simulink model "W02_pid"  (R2024b)
settings: Solver=ode4  StartTime=0  StopTime=T_final  FixedStep=h  RelTol=1e-3
StopFcn:
  | W02_plot;
values from neighbouring files (symbols this model uses):
  d_filtered = 1    [W02_0_setup.m]
  Kb = 2    [W02_0_setup.m]
  Kd = 4    [W02_0_setup.m]    (also in W02_E_integral.m; W02_I_tuning_by_hand.m = 1)
  Ki = 8    [W02_0_setup.m]
  Kp = 10    [W02_0_setup.m]    (also in W02_D_derivative.m; W02_E_integral.m; W02_I_tuning_by_hand.m = 5*k)
  Nf = 20    [W02_0_setup.m]    (also in W02_G_lowpass_filter.m = Nf(i))
  noise_std = 0    [W02_0_setup.m]
  noise_ts = 0.01    [W02_0_setup.m]
  pid_b = 2    [W02_0_setup.m]
  pid_k = 2    [W02_0_setup.m]
  pid_m = 1    [W02_0_setup.m]
  ref_filter = 0    [W02_0_setup.m]
  ref_Tf = 0.3    [W02_0_setup.m]
  t_step = 1    [W02_0_setup.m]
  tau_max = 1e6    (= 1000000)    [W02_0_setup.m]
  y_step = 1    [W02_0_setup.m]
libraries: slpidlib x1
settings Model: Creator=admin  LastModifiedBy=admin
settings DataIOCC: ReturnWorkspaceOutputs=off

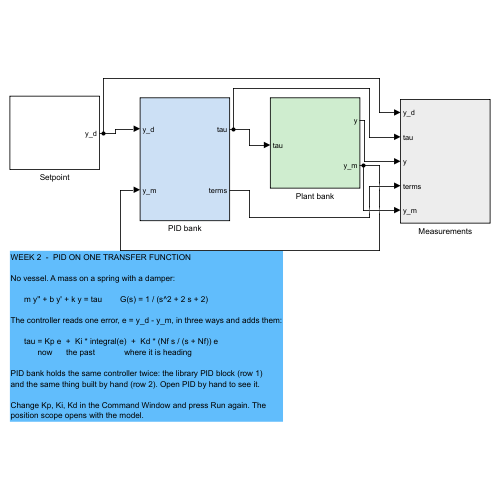
[thumbnail: Simulink's stored preview of the top-level diagram]
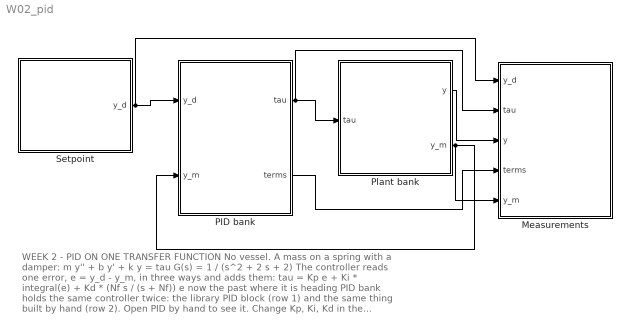
== system W02_pid ==
  note: WEEK 2  -  PID ON ONE TRANSFER FUNCTION
      |
      | No vessel. A mass on a spring with a damper:
      |
      |       m y'' + b y' + k y = tau        G(s) = 1 / (s^2 + 2 s + 2)
      |
      | The controller reads one error, e = y_d - y_m, in three ways and adds them:
      |
      |       tau = Kp e  +  Ki * integral(e)  +  Kd * (Nf s / (s + Nf)) e
      |             now      the past             where it is heading
      |
      | PID bank holds the same controller twice: the library PID block (row 1)
      | and the same thing built by hand (row 2). Open PID by hand to see it.
      |
      | Change Kp, Ki, Kd in the Command Window and press Run again. The
      | position scope opens with the model.
  Measurements : Subsystem
  PID bank : Subsystem
  Plant bank : Subsystem
  Setpoint : Subsystem
  wires:
  Setpoint/1(y_d) -> PID bank/1(y_d), Measurements/1(y_d)
  Plant bank/2(y_m) -> PID bank/2(y_m), Measurements/5(y_m)
  PID bank/1(tau) -> Plant bank/1(tau), Measurements/2(tau)
  Plant bank/1(y) -> Measurements/3(y)
  PID bank/2(terms) -> Measurements/4(terms)

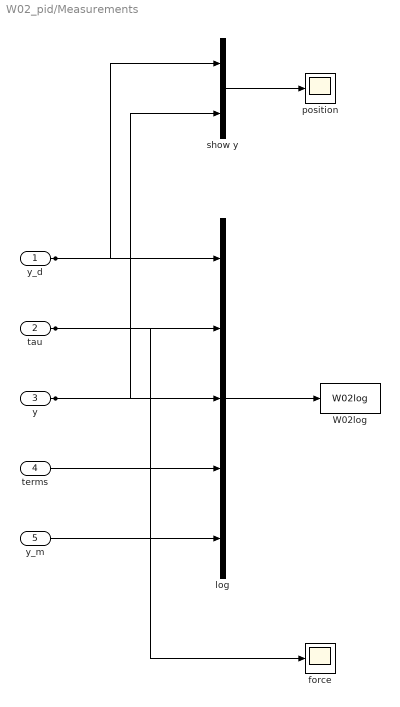
== system W02_pid/Measurements ==
  y_d : Inport
  tau : Inport  Port=2
  y : Inport  Port=3
  terms : Inport  Port=4
  y_m : Inport  Port=5
  W02log : ToWorkspace  VariableName=W02log  SaveFormat=Structure With Time  SampleTime=-1
  force : Scope
  log : Mux  Inputs=5
  position : Scope
  show y : Mux  Inputs=2
  wires:
  y_d/1 -> log/1, show y/1
  tau/1 -> log/2, force/1
  y/1 -> log/3, show y/2
  terms/1 -> log/4
  y_m/1 -> log/5
  log/1 -> W02log/1
  show y/1 -> position/1

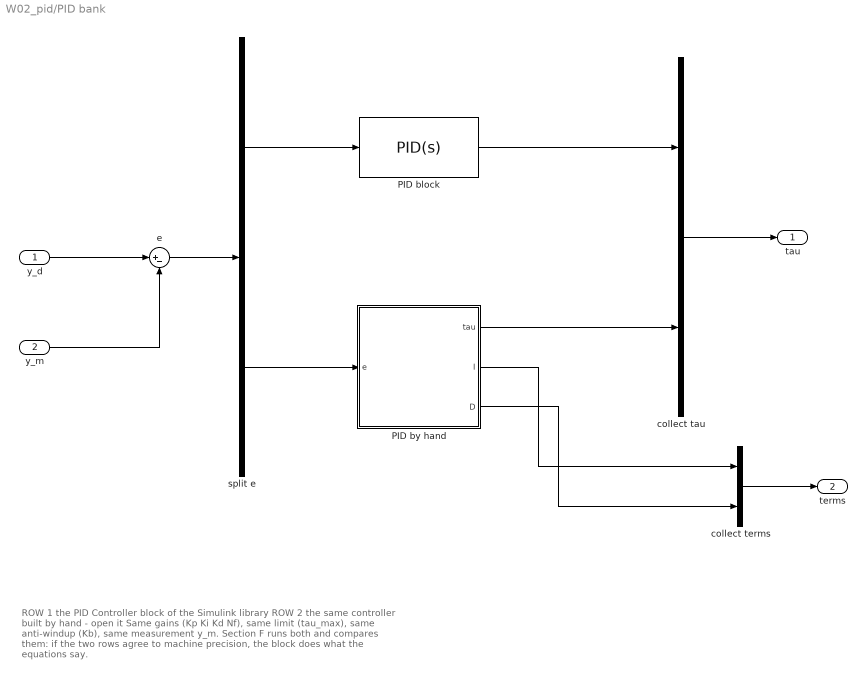
== system W02_pid/PID bank ==
  note: ROW 1  the PID Controller block of the Simulink library
      | ROW 2  the same controller built by hand - open it
      |
      | Same gains (Kp Ki Kd Nf), same limit (tau_max), same anti-windup (Kb),
      | same measurement y_m. Section F runs both and compares them: if the
      | two rows agree to machine precision, the block does what the equations say.
  y_d : Inport
  y_m : Inport  Port=2
  PID block : slpidlib/PID Controller  Controller=PID  Form=Parallel  TimeDomain=Continuous-time  UseExternalTs=off  SampleTime=-1  IntegratorMethod=Forward Euler  FilterMethod=Forward Euler  ControllerParametersSource=internal  P=Kp  I=Ki  UseKiTs=off  D=Kd  UseExternalDerivativeSource=off  N=Nf  UseFilter=on  TunerSelectOption=Transfer Function Based (PID Tuner App)  InitialConditionSource=internal  InitialConditionForIntegrator=0  InitialConditionForFilter=0  DifferentiatorICPrevScaledInput=0  ExternalReset=none  TrackingMode=off  Kt=1  LimitOutput=on  SatLimitsSource=internal  UpperSaturationLimit=tau_max  LowerSaturationLimit=-tau_max  LinearizeAsGain=on  AntiWindupMode=back-calculation  Kb=Kb  LimitIntegrator=off  UpperIntegratorSaturationLimit=inf  LowerIntegratorSaturationLimit=-inf  POutMin=[]  POutMax=[]  IOutMin=[]  IOutMax=[]  DOutMin=[]  DOutMax=[]  NOutMin=[]  NOutMax=[]  SumOutMin=[]  SumOutMax=[]  SaturationOutMin=[]  SaturationOutMax=[]  PParamMin=[]  PParamMax=[]  IParamMin=[]  IParamMax=[]  DParamMin=[]  DParamMax=[]  NParamMin=[]  NParamMax=[]  KbParamMin=[]  KbParamMax=[]  KtParamMin=[]  KtParamMax=[]  KbOutMin=[]  KbOutMax=[]  KtOutMin=[]  KtOutMax=[]  IntegratorOutMin=[]  IntegratorOutMax=[]  FilterOutMin=[]  FilterOutMax=[]  SumI1OutMin=[]  SumI1OutMax=[]  SumI2OutMin=[]  SumI2OutMax=[]  SumI3OutMin=[]  SumI3OutMax=[]  SumI4OutMin=[]  SumI4OutMax=[]  SumDOutMin=[]  SumDOutMax=[]  DifferentiatorOutMin=[]  DifferentiatorOutMax=[]  FilterDiffOutCoefMin=[]  FilterDiffOutCoefMax=[]  ReciprocalOutMin=[]  ReciprocalOutMax=[]  SumDenOutMin=[]  SumDenOutMax=[]  SumNumOutMin=[]  SumNumOutMax=[]  DivideOutMin=[]  DivideOutMax=[]  UdiffTsProdOutMin=[]  UdiffTsProdOutMax=[]  NTsProdOutMin=[]  NTsProdOutMax=[]  UintegralTsProdOutMin=[]  UintegralTsProdOutMax=[]  UngainTsProdOutMin=[]  UngainTsProdOutMax=[]  ClampingZeroOutDataTypeStr=Inherit: Inherit via back propagation  ClampingZeroOutMin=[]  ClampingZeroOutMax=[]  FilterDenConstantOutDataTypeStr=Inherit: Inherit via back propagation  FilterDenConstantOutMin=[]  FilterDenConstantOutMax=[]  PCopyOutDataTypeStr=Inherit: Inherit via back propagation  PCopyOutMin=[]  PCopyOutMax=[]  NCopyOutDataTypeStr=Inherit: Inherit via back propagation  NCopyOutMin=[]  NCopyOutMax=[]  IntegratorContinuousStateAttributes=''  IntegratorStateMustResolveToSignalObject=off  IntegratorRTWStateStorageClass=Auto  FilterContinuousStateAttributes=''  FilterStateMustResolveToSignalObject=off  FilterRTWStateStorageClass=Auto  ParallelPVariant=InternalParameters  IdealPVariant=Disabled  IVariant=InternalParameters  DVariant=InternalParameters  IntegratorVariant=Continuous  SatVariant=Enabled  AWVariant=BackCalculation  PCopyVariant=Disabled  TRVariant=Disabled  FdbkBlocksVariant=Forward  IdealPFdbkVariant=Disabled  SatFdbkVariant=Disabled  DerivativeFilterVariant=ContFilter  NVariant=InternalParameters  NCopyVariant=Disabled  FilterICVariant=InternalICsFilter  IntegratorICVariant=InternalICs  ExternalResetVariant=Disabled  TRSumVariant=Passthrough  SumFdbkVariant=Disabled  SumVariant=Sum_PID  TsampFilterVariant=InternalTs  TsampNgainVariant=Passthrough  TsampIntegralVariant=Disabled_SignalSpec  ExternalSaturationOutDataTypeStr=Inherit: Same as second input  DerivativeSourceVariant=ErrorSignal  PreIntVariant=InternalPreInt
  PID by hand : Subsystem
  collect tau : Mux  Inputs=2
  collect terms : Mux  Inputs=2
  e : Sum  Inputs=|+-
  split e : Demux  Outputs=2
  tau : Outport
  terms : Outport  Port=2
  wires:
  y_d/1 -> e/1
  y_m/1 -> e/2
  e/1 -> split e/1
  split e/1 -> PID block/1
  split e/2 -> PID by hand/1(e)
  PID block/1 -> collect tau/1
  PID by hand/1(tau) -> collect tau/2
  collect tau/1 -> tau/1
  PID by hand/2(I) -> collect terms/1
  PID by hand/3(D) -> collect terms/2
  collect terms/1 -> terms/1

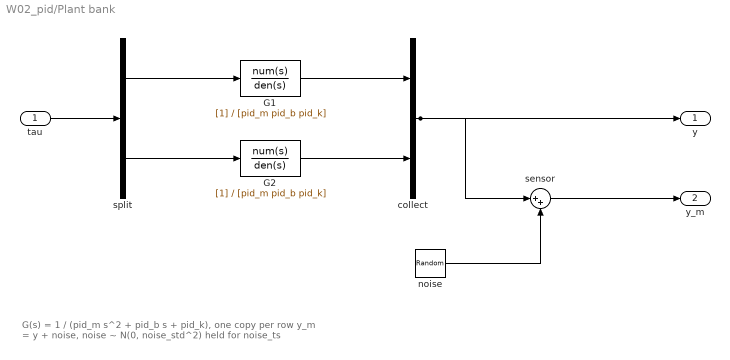
== system W02_pid/Plant bank ==
  note: G(s) = 1 / (pid_m s^2 + pid_b s + pid_k),  one copy per row
      | y_m  = y + noise,  noise ~ N(0, noise_std^2) held for noise_ts
  tau : Inport
  G1 : TransferFcn  Denominator=[pid_m pid_b pid_k]
  G2 : TransferFcn  Denominator=[pid_m pid_b pid_k]
  collect : Mux  Inputs=2
  noise : RandomNumber  Variance=noise_std^2  Seed=23341  SampleTime=noise_ts
  sensor : Sum  Inputs=|++
  split : Demux  Outputs=2
  y : Outport
  y_m : Outport  Port=2
  wires:
  tau/1 -> split/1
  split/1 -> G1/1
  G1/1 -> collect/1
  split/2 -> G2/1
  G2/1 -> collect/2
  collect/1 -> y/1, sensor/1
  noise/1 -> sensor/2
  sensor/1 -> y_m/1

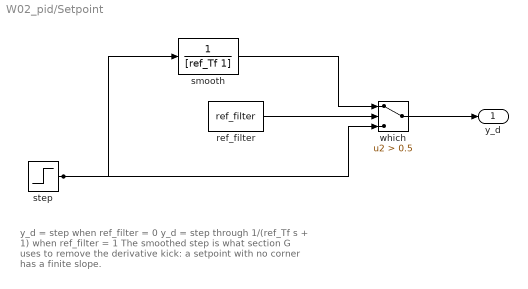
== system W02_pid/Setpoint ==
  note: y_d = step                          when ref_filter = 0
      | y_d = step through 1/(ref_Tf s + 1)  when ref_filter = 1
      |
      | The smoothed step is what section G uses to remove the
      | derivative kick: a setpoint with no corner has a finite slope.
  ref_filter : Constant  Value=ref_filter
  smooth : TransferFcn  Denominator=[ref_Tf 1]
  step : Step  Time=t_step  After=y_step  SampleTime=0
  which : Switch  Criteria=u2 > Threshold  Threshold=0.5  SaturateOnIntegerOverflow=off  InputSameDT=off
  y_d : Outport
  wires:
  step/1 -> smooth/1, which/3
  smooth/1 -> which/1
  ref_filter/1 -> which/2
  which/1 -> y_d/1

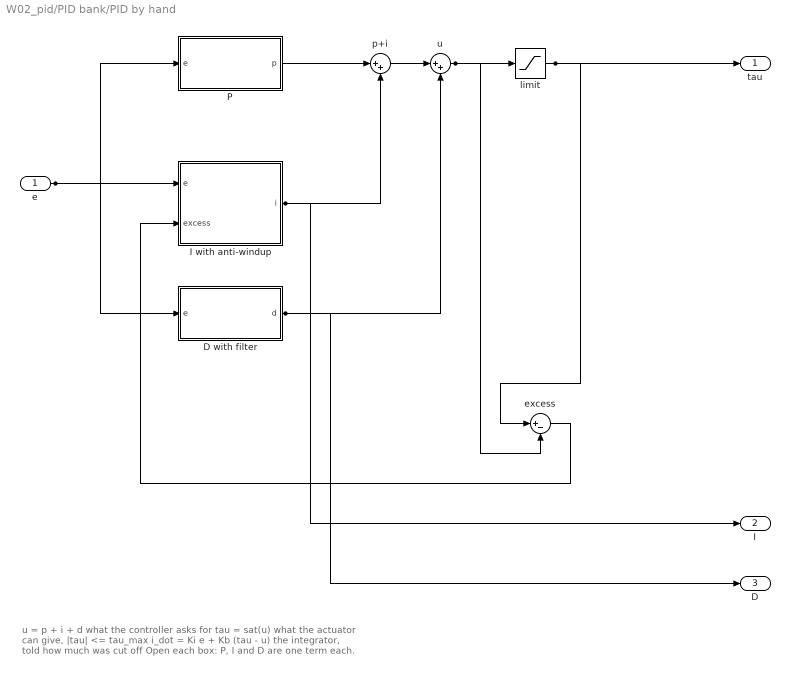
== system W02_pid/PID bank/PID by hand ==
  note: u     = p + i + d          what the controller asks for
      | tau   = sat(u)             what the actuator can give, |tau| <= tau_max
      | i_dot = Ki e + Kb (tau - u)   the integrator, told how much was cut off
      |
      | Open each box: P, I and D are one term each.
  e : Inport
  D with filter : Subsystem
  I with anti-windup : Subsystem
  P : Subsystem
  excess : Sum  Inputs=|+-
  limit : Saturate  UpperLimit=tau_max  LowerLimit=-tau_max
  p+i : Sum  Inputs=|++
  u : Sum  Inputs=|++
  tau : Outport
  I : Outport  Port=2
  D : Outport  Port=3
  wires:
  e/1 -> P/1(e), I with anti-windup/1(e), D with filter/1(e)
  P/1(p) -> p+i/1
  I with anti-windup/1(i) -> p+i/2, I/1
  D with filter/1(d) -> u/2, D/1
  p+i/1 -> u/1
  u/1 -> limit/1, excess/2
  limit/1 -> tau/1, excess/1
  excess/1 -> I with anti-windup/2(excess)

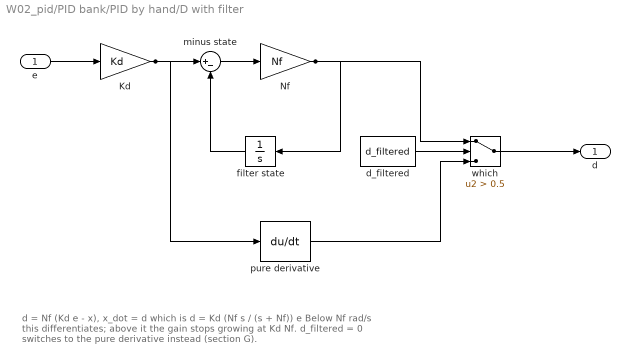
== system W02_pid/PID bank/PID by hand/D with filter ==
  note: d = Nf (Kd e - x),  x_dot = d        which is   d = Kd (Nf s / (s + Nf)) e
      |
      | Below Nf rad/s this differentiates; above it the gain stops growing at Kd Nf.
      | d_filtered = 0 switches to the pure derivative instead (section G).
  e : Inport
  Kd : Gain  Gain=Kd
  Nf : Gain  Gain=Nf
  d_filtered : Constant  Value=d_filtered
  filter state : Integrator
  minus state : Sum  Inputs=|+-
  pure derivative : Derivative
  which : Switch  Criteria=u2 > Threshold  Threshold=0.5  SaturateOnIntegerOverflow=off  InputSameDT=off
  d : Outport
  wires:
  e/1 -> Kd/1
  Kd/1 -> minus state/1, pure derivative/1
  minus state/1 -> Nf/1
  Nf/1 -> which/1, filter state/1
  filter state/1 -> minus state/2
  d_filtered/1 -> which/2
  pure derivative/1 -> which/3
  which/1 -> d/1

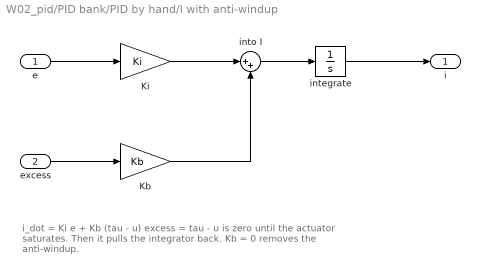
== system W02_pid/PID bank/PID by hand/I with anti-windup ==
  note: i_dot = Ki e + Kb (tau - u)
      |
      | excess = tau - u is zero until the actuator saturates. Then it pulls
      | the integrator back. Kb = 0 removes the anti-windup.
  e : Inport
  excess : Inport  Port=2
  Kb : Gain  Gain=Kb
  Ki : Gain  Gain=Ki
  integrate : Integrator
  into I : Sum  Inputs=|++
  i : Outport
  wires:
  e/1 -> Ki/1
  excess/1 -> Kb/1
  Ki/1 -> into I/1
  Kb/1 -> into I/2
  into I/1 -> integrate/1
  integrate/1 -> i/1

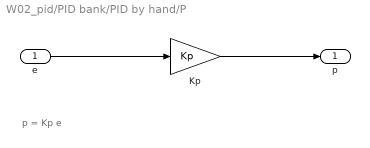
== system W02_pid/PID bank/PID by hand/P ==
  note: p = Kp e
  e : Inport
  Kp : Gain  Gain=Kp
  p : Outport
  wires:
  e/1 -> Kp/1
  Kp/1 -> p/1
